simulink model "fixlib"  (Simulink 6.2)
settings: Solver=ode45  SolverMode=SingleTasking  StartTime=0.0  StopTime=10.0  RelTol=1e-3  AbsTol=1e-6
undefined symbols (not defined in the file or in its folder): k
settings Model: Creator=jacobs  LastModifiedBy=jacobs  ExtModeAutoUpdateStatusClock=off
settings DataIOCC: LimitDataPoints=off
settings OptimizationCC: BlockReduction=off  BooleanDataType=off
settings HardwareCC: TargetUnknown=on
settings GRTTargetCC: ModelReferenceCompliant=off  MatFileLogging=off

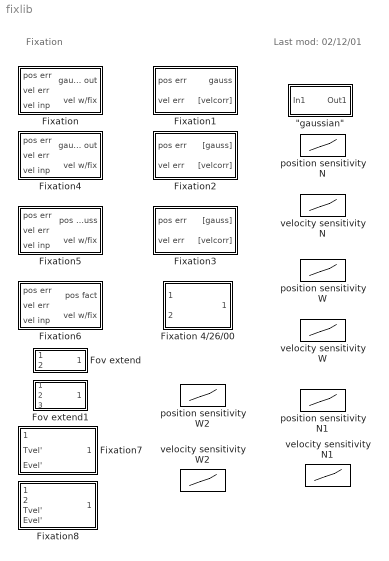
== system fixlib ==
  note: Last mod: 02/12/01
  note: Fixation
  "\"gaussian\"" : Subsystem
      mask Display: disp('"gaussian"')
  Fixation : Subsystem
  "Fixation 4/26/00 " : Subsystem
  Fixation1 : Subsystem
  Fixation2 : Subsystem
  Fixation3 : Subsystem
  Fixation4 : Subsystem
  Fixation5 : Subsystem
  Fixation6 : Subsystem
  Fixation7 : Subsystem
      mask Display: disp('Fixation')
  Fixation8 : Subsystem
      mask Display: disp('Fixation')
  Fov extend : Subsystem
      mask Display: disp('Fov Exten')
  Fov extend1 : Subsystem
      mask Display: disp('Fov Exten')
  position sensitivity N : Lookup  InputValues="[-5 -2  -1 -0.5   0.5   1    2    5]"  OutputValues="[  0    0   0.5   1      1   0.5   0   0 ]"  SaturateOnIntegerOverflow=on
  position sensitivity N1 : Lookup  InputValues="[-2  -1 -0.5 -0.25   0.25   0.5   1  2]"  OutputValues="[  0    0   .5   1      1   .5   0   0 ]"  SaturateOnIntegerOverflow=on
  position sensitivity W : Lookup  InputValues="[-5 -2  -1 -0.5   0.5   1    2    5]"  OutputValues="[ 0   0.5    1     1      1     1    0.5  0]"  SaturateOnIntegerOverflow=on
  position sensitivity W2 : Lookup  InputValues="[-5 -2  -1 -0.5   0.5   1    2    5]"  OutputValues="[ 0   0.125    0.5     1      1     0.5    0.125  0]"  SaturateOnIntegerOverflow=on
  velocity sensitivity N : Lookup  InputValues="[-30 -15   -8  -4   4     8  15  30]"  OutputValues="[  0      0      0.5    1   1  0.5   0   0 ]"  SaturateOnIntegerOverflow=on
  velocity sensitivity N1 : Lookup  InputValues="[-20 -16  -12   -6  -4  4   6   12  16 20]"  OutputValues="[0 0   0.1    0.3    1   1   0.3  0.1   0 0]"  SaturateOnIntegerOverflow=on
  velocity sensitivity W : Lookup  InputValues="[-30 -15   -8  -4   4     8  15  30]"  OutputValues="[0  0.5   1    1    1    1   0.5  0]"  SaturateOnIntegerOverflow=on
  velocity sensitivity W2 : Lookup  InputValues="[-30 -15   -8  -4   4     8  15  30]"  OutputValues="[0  0.125   0.5    1    1    0.5   0.125  0]"  SaturateOnIntegerOverflow=on

== system fixlib/"gaussian" ==
  note: calculates 1-e^(n*x*x) which is gaussian-like.
  In1 : Inport  Port=1  LatchInput=off
  Math Function : Math  SaturateOnIntegerOverflow=on
  Product : Product  Inputs=3  SaturateOnIntegerOverflow=on  RndMeth=Zero  InputSameDT=on
  n : Constant  Value=-1/4
  Out1 : Outport  InitialOutput=0
  wires:
  n/1 -> Product/3
  In1/1 -> Product/2, Product/1
  Product/1 -> Math Function/1
  Math Function/1 -> Out1/1

== system fixlib/Fixation ==
  note: This should have the effect of reducing the high velocity error (due
      | to CN oscillation or other sources) enough to permit an extension of
      | the foveation period.
  note: This factor is used (with an additional gain factor) to scale the velocity error,
      | which is then subtracted from the velocity signal that is sent from the
      | common neural integrator to the ocular motor neurons.
  note: Positional error is passed through a gaussian-like function whose greatest
      | response occurs between +/-0.5 deg (approx), corresponding to the sensitivity
      | of the fovea.
  note: Last mod: 04/19/00
  note: Fixation
  pos err : Inport  Port=1  LatchInput=off
  vel err : Inport  Port=2  LatchInput=off
  vel inp : Inport  Port=3  LatchInput=off
  "\"gaussian\"" : Subsystem
      mask Display: disp('"gaussian"')
  "\"gaussian\" gain" : Constant  Value=.5
  Product : Product  Inputs=3  SaturateOnIntegerOverflow=on  RndMeth=Zero  InputSameDT=on
  Sum : Sum  Inputs=-+  SaturateOnIntegerOverflow=on  InputSameDT=on
  gauss out : Outport  InitialOutput=0
  vel w/fix : Outport  Port=2  InitialOutput=0
  wires:
  "\"gaussian\" gain"/1 -> Product/2
  "\"gaussian\""/1(Out1) -> gauss out/1, Product/1
  pos err/1 -> "\"gaussian\""/1(In1)
  vel err/1 -> Product/3
  Product/1 -> Sum/1
  vel inp/1 -> Sum/2
  Sum/1 -> vel w/fix/1

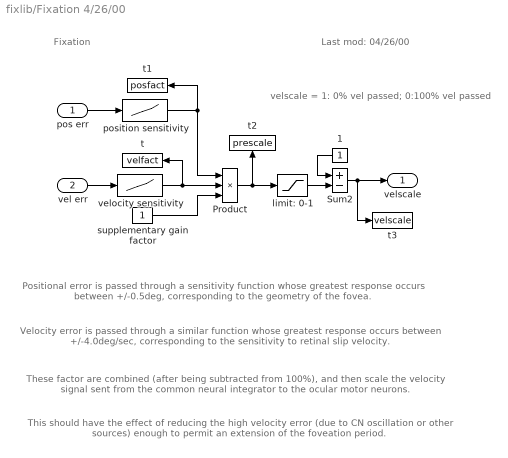
== system fixlib/Fixation 4/26/00  ==
  note: velscale =
      | 1: 0% vel passed;
      | 0:100% vel passed
  note: Velocity error is passed through a similar function whose greatest
      | response occurs between +/-4.0deg/sec, corresponding to the sensitivity
      | to retinal slip velocity.
  note: This should have the effect of reducing the high velocity error (due
      | to CN oscillation or other sources) enough to permit an extension of
      | the foveation period.
  note: These factor are combined (after being subtracted from 100%),
      | and then scale the velocity signal sent from the
      | common neural integrator to the ocular motor neurons.
  note: Positional error is passed through a sensitivity function whose greatest
      | response occurs between +/-0.5deg, corresponding to the geometry
      | of the fovea.
  note: Last mod: 04/26/00
  note: Fixation
  pos err : Inport  Port=1  LatchInput=off
  vel err : Inport  Port=2  LatchInput=off
  1 : Constant  Orientation=left
  Product : Product  Inputs=3  SaturateOnIntegerOverflow=on  RndMeth=Zero  InputSameDT=on
  Sum2 : Sum  Inputs=+-  SaturateOnIntegerOverflow=on  InputSameDT=on
  limit: 0-1 : Saturate  UpperLimit=1  LowerLimit=0
  position sensitivity : Lookup  InputValues="[-5 -2    -1  -0.5   0.5     1    2    5]"  OutputValues="[  0    0   0.25   1      1   0.25   0   0 ]"  SaturateOnIntegerOverflow=on
  supplementary gain factor : Constant
  t : ToWorkspace  VariableName=velfact  SaveFormat=Array
      mask init:
      | global t
      settings: MaxDataPoints=100000
  t1 : ToWorkspace  VariableName=posfact  SaveFormat=Array
      mask init:
      | global t
      settings: MaxDataPoints=100000
  t2 : ToWorkspace  VariableName=prescale  SaveFormat=Array
      mask init:
      | global t
      settings: Orientation=up  MaxDataPoints=100000
  t3 : ToWorkspace  VariableName=velscale  SaveFormat=Array
      mask init:
      | global t
      settings: MaxDataPoints=100000
  velocity sensitivity : Lookup  InputValues="[-30 -15    -8   -4    4     8    15  30]"  OutputValues="[  0      0      0.25    1   1  0.25   0   0 ]"  SaturateOnIntegerOverflow=on
  velscale : Outport  InitialOutput=0
  wires:
  Sum2/1 -> t3/1, velscale/1
  limit: 0-1/1 -> Sum2/2
  1/1 -> Sum2/1
  position sensitivity/1 -> Product/1, t1/1
  pos err/1 -> position sensitivity/1
  Product/1 -> limit: 0-1/1, t2/1
  velocity sensitivity/1 -> t/1, Product/2
  supplementary gain factor/1 -> Product/3
  vel err/1 -> velocity sensitivity/1

== system fixlib/Fixation1 ==
  note: velocity
      | correction
  note: This should have the effect of reducing the high velocity error (due
      | to CN oscillation or other sources) enough to permit an extension of
      | the foveation period.
  note: This factor is used (with an additional gain factor) to scale the velocity error,
      | which will then subtracted from the velocity signal that is sent from the
      | common neural integrator to the ocular motor neurons.
  note: Positional error is passed through a gaussian-like function whose greatest
      | response occurs between +/-0.5 deg (approx), corresponding to the sensitivity
      | of the fovea.
  note: Last mod: 04/19/00
  note: Fixation
  pos err : Inport  Port=1  LatchInput=off
  vel err : Inport  Port=2  LatchInput=off
  "\"gaussian\"" : Subsystem
      mask Display: disp('"gaussian"')
  "\"gaussian\" gain" : Constant  Value=.5
  Product : Product  Inputs=3  SaturateOnIntegerOverflow=on  RndMeth=Zero  InputSameDT=on
  To Workspace30 : ToWorkspace  VariableName=velcorr  SaveFormat=Array
      settings: MaxDataPoints=10000
  gauss : Outport  InitialOutput=0
  "[velcorr]" : Outport  Port=2  InitialOutput=0
  wires:
  Product/1 -> To Workspace30/1, "[velcorr]"/1
  "\"gaussian\" gain"/1 -> Product/2
  "\"gaussian\""/1(Out1) -> gauss/1, Product/1
  pos err/1 -> "\"gaussian\""/1(In1)
  vel err/1 -> Product/3

== system fixlib/Fixation2 ==
  note: [tpstar]
  note: [svpr]
  note: velocity
      | correction
  note: This should have the effect of reducing the high velocity error (due
      | to CN oscillation or other sources) enough to permit an extension of
      | the foveation period.
  note: This factor is used (with an additional gain factor) to scale the velocity error,
      | which will then subtracted from the velocity signal that is sent from the
      | common neural integrator to the ocular motor neurons.
  note: Positional error is passed through a gaussian-like function whose greatest
      | response occurs between +/-0.5 deg (approx), corresponding to the sensitivity
      | of the fovea.
  note: Last mod: 04/21/00
  note: Fixation
  pos err : Inport  Port=1  LatchInput=off
  vel err : Inport  Port=2  LatchInput=off
  "\"gaussian\"" : Subsystem
      mask Display: disp('"gaussian"')
  "\"gaussian\" gain" : Constant  Value=.5
  Product : Product  Inputs=3  SaturateOnIntegerOverflow=on  RndMeth=Zero  InputSameDT=on
  Product1 : Product  SaturateOnIntegerOverflow=on  RndMeth=Zero  InputSameDT=on
  To Workspace30 : ToWorkspace  VariableName=velcorr  SaveFormat=Array
      settings: MaxDataPoints=10000
  k : Constant  Value=k
  "[gauss]" : Outport  InitialOutput=0
  "[velcorr]" : Outport  Port=2  InitialOutput=0
  wires:
  k/1 -> Product/3
  Product/1 -> To Workspace30/1, "[velcorr]"/1
  Product1/1 -> Product/1, "[gauss]"/1
  "\"gaussian\" gain"/1 -> Product1/2
  "\"gaussian\""/1(Out1) -> Product1/1
  pos err/1 -> "\"gaussian\""/1(In1)
  vel err/1 -> Product/2

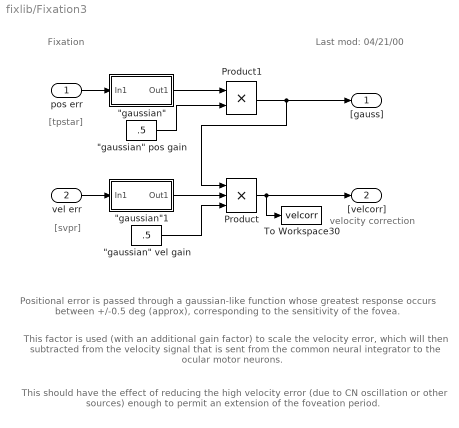
== system fixlib/Fixation3 ==
  note: [tpstar]
  note: [svpr]
  note: velocity
      | correction
  note: This should have the effect of reducing the high velocity error (due
      | to CN oscillation or other sources) enough to permit an extension of
      | the foveation period.
  note: This factor is used (with an additional gain factor) to scale the velocity error,
      | which will then subtracted from the velocity signal that is sent from the
      | common neural integrator to the ocular motor neurons.
  note: Positional error is passed through a gaussian-like function whose greatest
      | response occurs between +/-0.5 deg (approx), corresponding to the sensitivity
      | of the fovea.
  note: Last mod: 04/21/00
  note: Fixation
  pos err : Inport  Port=1  LatchInput=off
  vel err : Inport  Port=2  LatchInput=off
  "\"gaussian\"" : Subsystem
      mask Display: disp('"gaussian"')
  "\"gaussian\" pos gain" : Constant  Value=.5
  "\"gaussian\" vel gain" : Constant  Value=.5
  "\"gaussian\"1" : Subsystem
      mask Display: disp('"gaussian"')
  Product : Product  Inputs=3  SaturateOnIntegerOverflow=on  RndMeth=Zero  InputSameDT=on
  Product1 : Product  SaturateOnIntegerOverflow=on  RndMeth=Zero  InputSameDT=on
  To Workspace30 : ToWorkspace  VariableName=velcorr  SaveFormat=Array
      settings: MaxDataPoints=10000
  "[gauss]" : Outport  InitialOutput=0
  "[velcorr]" : Outport  Port=2  InitialOutput=0
  wires:
  "\"gaussian\" vel gain"/1 -> Product/3
  Product/1 -> To Workspace30/1, "[velcorr]"/1
  "\"gaussian\"1"/1(Out1) -> Product/2
  vel err/1 -> "\"gaussian\"1"/1(In1)
  Product1/1 -> Product/1, "[gauss]"/1
  "\"gaussian\" pos gain"/1 -> Product1/2
  "\"gaussian\""/1(Out1) -> Product1/1
  pos err/1 -> "\"gaussian\""/1(In1)

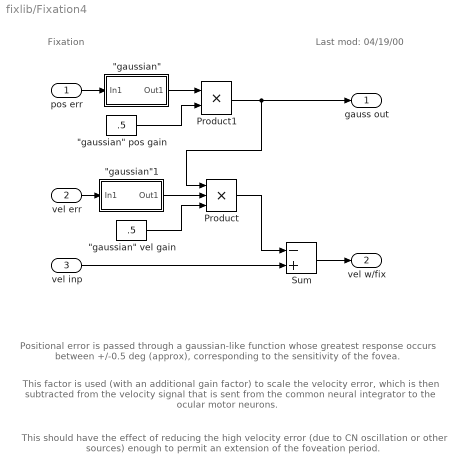
== system fixlib/Fixation4 ==
  note: This should have the effect of reducing the high velocity error (due
      | to CN oscillation or other sources) enough to permit an extension of
      | the foveation period.
  note: This factor is used (with an additional gain factor) to scale the velocity error,
      | which is then subtracted from the velocity signal that is sent from the
      | common neural integrator to the ocular motor neurons.
  note: Positional error is passed through a gaussian-like function whose greatest
      | response occurs between +/-0.5 deg (approx), corresponding to the sensitivity
      | of the fovea.
  note: Last mod: 04/19/00
  note: Fixation
  pos err : Inport  Port=1  LatchInput=off
  vel err : Inport  Port=2  LatchInput=off
  vel inp : Inport  Port=3  LatchInput=off
  "\"gaussian\"" : Subsystem
      mask Display: disp('"gaussian"')
  "\"gaussian\" pos gain" : Constant  Value=.5
  "\"gaussian\" vel gain" : Constant  Value=.5
  "\"gaussian\"1" : Subsystem
      mask Display: disp('"gaussian"')
  Product : Product  Inputs=3  SaturateOnIntegerOverflow=on  RndMeth=Zero  InputSameDT=on
  Product1 : Product  SaturateOnIntegerOverflow=on  RndMeth=Zero  InputSameDT=on
  Sum : Sum  Inputs=-+  SaturateOnIntegerOverflow=on  InputSameDT=on
  gauss out : Outport  InitialOutput=0
  vel w/fix : Outport  Port=2  InitialOutput=0
  wires:
  "\"gaussian\" vel gain"/1 -> Product/3
  vel inp/1 -> Sum/2
  Sum/1 -> vel w/fix/1
  "\"gaussian\"1"/1(Out1) -> Product/2
  vel err/1 -> "\"gaussian\"1"/1(In1)
  Product1/1 -> Product/1, gauss out/1
  "\"gaussian\" pos gain"/1 -> Product1/2
  "\"gaussian\""/1(Out1) -> Product1/1
  Product/1 -> Sum/1
  pos err/1 -> "\"gaussian\""/1(In1)

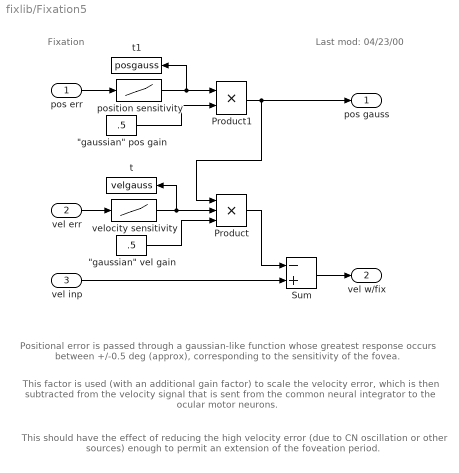
== system fixlib/Fixation5 ==
  note: This should have the effect of reducing the high velocity error (due
      | to CN oscillation or other sources) enough to permit an extension of
      | the foveation period.
  note: This factor is used (with an additional gain factor) to scale the velocity error,
      | which is then subtracted from the velocity signal that is sent from the
      | common neural integrator to the ocular motor neurons.
  note: Positional error is passed through a gaussian-like function whose greatest
      | response occurs between +/-0.5 deg (approx), corresponding to the sensitivity
      | of the fovea.
  note: Last mod: 04/23/00
  note: Fixation
  pos err : Inport  Port=1  LatchInput=off
  vel err : Inport  Port=2  LatchInput=off
  vel inp : Inport  Port=3  LatchInput=off
  "\"gaussian\" pos gain" : Constant  Value=.5
  "\"gaussian\" vel gain" : Constant  Value=.5
  Product : Product  Inputs=3  SaturateOnIntegerOverflow=on  RndMeth=Zero  InputSameDT=on
  Product1 : Product  SaturateOnIntegerOverflow=on  RndMeth=Zero  InputSameDT=on
  Sum : Sum  Inputs=-+  SaturateOnIntegerOverflow=on  InputSameDT=on
  position sensitivity : Lookup  InputValues="[-5 -2  -1 -0.5   0.5   1    2    5]"  OutputValues="[  0    0   0.5   1      1   0.5   0   0 ]"  SaturateOnIntegerOverflow=on
  t : ToWorkspace  VariableName=velgauss  SaveFormat=Array
      mask init:
      | global t
      settings: MaxDataPoints=100000
  t1 : ToWorkspace  VariableName=posgauss  SaveFormat=Array
      mask init:
      | global t
      settings: MaxDataPoints=100000
  velocity sensitivity : Lookup  InputValues="[-30 -15   -8  -4   4     8  15  30]"  OutputValues="[  0      0      0.5    1   1  0.5   0   0 ]"  SaturateOnIntegerOverflow=on
  pos gauss : Outport  InitialOutput=0
  vel w/fix : Outport  Port=2  InitialOutput=0
  wires:
  position sensitivity/1 -> t1/1, Product1/1
  velocity sensitivity/1 -> t/1, Product/2
  "\"gaussian\" vel gain"/1 -> Product/3
  vel inp/1 -> Sum/2
  Sum/1 -> vel w/fix/1
  vel err/1 -> velocity sensitivity/1
  Product/1 -> Sum/1
  Product1/1 -> Product/1, pos gauss/1
  "\"gaussian\" pos gain"/1 -> Product1/2
  pos err/1 -> position sensitivity/1

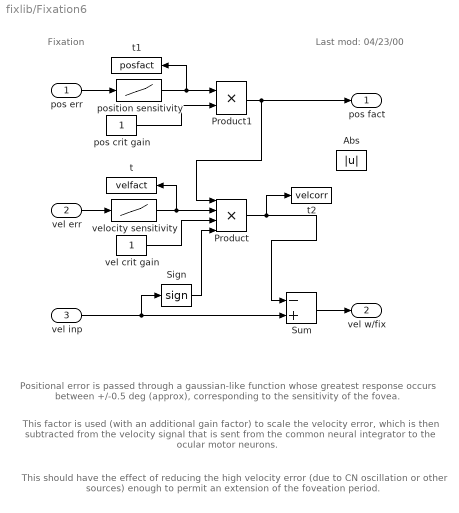
== system fixlib/Fixation6 ==
  note: This should have the effect of reducing the high velocity error (due
      | to CN oscillation or other sources) enough to permit an extension of
      | the foveation period.
  note: This factor is used (with an additional gain factor) to scale the velocity error,
      | which is then subtracted from the velocity signal that is sent from the
      | common neural integrator to the ocular motor neurons.
  note: Positional error is passed through a gaussian-like function whose greatest
      | response occurs between +/-0.5 deg (approx), corresponding to the sensitivity
      | of the fovea.
  note: Last mod: 04/23/00
  note: Fixation
  pos err : Inport  Port=1  LatchInput=off
  vel err : Inport  Port=2  LatchInput=off
  vel inp : Inport  Port=3  LatchInput=off
  Abs : Abs  SaturateOnIntegerOverflow=on
  Product : Product  Inputs=4  SaturateOnIntegerOverflow=on  RndMeth=Zero  InputSameDT=on
  Product1 : Product  SaturateOnIntegerOverflow=on  RndMeth=Zero  InputSameDT=on
  Sign : Signum
  Sum : Sum  Inputs=-+  SaturateOnIntegerOverflow=on  InputSameDT=on
  pos crit gain : Constant
  position sensitivity : Lookup  InputValues="[-5 -2  -1 -0.5   0.5   1    2    5]"  OutputValues="[  0    0   0.5   1      1   0.5   0   0 ]"  SaturateOnIntegerOverflow=on
  t : ToWorkspace  VariableName=velfact  SaveFormat=Array
      mask init:
      | global t
      settings: MaxDataPoints=100000
  t1 : ToWorkspace  VariableName=posfact  SaveFormat=Array
      mask init:
      | global t
      settings: MaxDataPoints=100000
  t2 : ToWorkspace  VariableName=velcorr  SaveFormat=Array
      mask init:
      | global t
      settings: MaxDataPoints=100000
  vel crit gain : Constant
  velocity sensitivity : Lookup  InputValues="[-30 -15   -8  -4   4     8  15  30]"  OutputValues="[  0      0      0.5    1   1  0.5   0   0 ]"  SaturateOnIntegerOverflow=on
  pos fact : Outport  InitialOutput=0
  vel w/fix : Outport  Port=2  InitialOutput=0
  wires:
  Product/1 -> t2/1, Sum/1
  Sign/1 -> Product/4
  vel inp/1 -> Sign/1, Sum/2
  Sum/1 -> vel w/fix/1
  position sensitivity/1 -> t1/1, Product1/1
  velocity sensitivity/1 -> t/1, Product/2
  vel crit gain/1 -> Product/3
  vel err/1 -> velocity sensitivity/1
  Product1/1 -> Product/1, pos fact/1
  pos crit gain/1 -> Product1/2
  pos err/1 -> position sensitivity/1

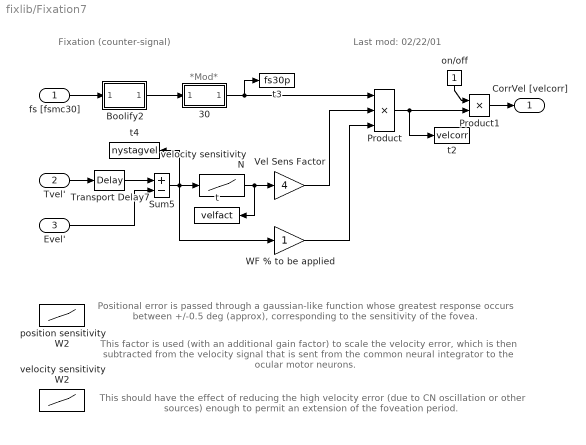
== system fixlib/Fixation7 ==
  note: *Mod*
  note: This should have the effect of reducing the high velocity error (due
      | to CN oscillation or other sources) enough to permit an extension of
      | the foveation period.
  note: This factor is used (with an additional gain factor) to scale the velocity error,
      | which is then subtracted from the velocity signal that is sent from the
      | common neural integrator to the ocular motor neurons.
  note: Positional error is passed through a gaussian-like function whose greatest
      | response occurs between +/-0.5 deg (approx), corresponding to the sensitivity
      | of the fovea.
  note: Last mod: 02/22/01
  note: Fixation (counter-signal)
  fs [fsmc30] : Inport  Port=1  LatchInput=off
  Tvel' : Inport  Port=2  LatchInput=off
  Evel' : Inport  Port=3  LatchInput=off
  "30 " : Subsystem  mask{prolong=30}
      mask prompts: prolong "Prolong pulse by?  (msec)"
      mask Display: disp('prolong')
  Boolify2 : Subsystem
      mask Display: disp('Boolify')
  Product : Product  Inputs=3  SaturateOnIntegerOverflow=on  RndMeth=Zero  InputSameDT=on
  Product1 : Product  SaturateOnIntegerOverflow=on  RndMeth=Zero  InputSameDT=on
  Sum5 : Sum  Inputs=+-  SaturateOnIntegerOverflow=on  InputSameDT=on
  Transport Delay7 : TransportDelay  DelayTime=0.050
      mask Display: disp('50ms')
  Vel Sens Factor : Gain  Gain=4  SaturateOnIntegerOverflow=on
  WF % to be applied : Gain  SaturateOnIntegerOverflow=on
  on/off : Constant  Orientation=down
  position sensitivity W2 : Lookup  InputValues="[-5 -2  -1 -0.5   0.5   1    2    5]"  OutputValues="[ 0   0.125    0.5     1      1     0.5    0.125  0]"  SaturateOnIntegerOverflow=on
  t : ToWorkspace  VariableName=velfact  SaveFormat=Array
      mask init:
      | global t
      settings: MaxDataPoints=100000
  t2 : ToWorkspace  VariableName=velcorr  SaveFormat=Array
      mask init:
      | global t
      settings: MaxDataPoints=100000
  t3 : ToWorkspace  VariableName=fs30p  SaveFormat=Array
      mask init:
      | global t
      settings: MaxDataPoints=100000
  t4 : ToWorkspace  VariableName=nystagvel  SaveFormat=Array
      mask init:
      | global t
      settings: MaxDataPoints=100000
  velocity sensitivity N : Lookup  InputValues="[-20 -16  -12   -6  -4  4   6   12  16 20]"  OutputValues="[0 0   0.1    0.3    1   1   0.3  0.1   0 0]"  SaturateOnIntegerOverflow=on
  velocity sensitivity W2 : Lookup  InputValues="[-30 -15   -8  -4   4     8  15  30]"  OutputValues="[0  0.125   0.5    1    1    0.5   0.125  0]"  SaturateOnIntegerOverflow=on
  " CorrVel [velcorr]" : Outport  InitialOutput=0
  wires:
  Vel Sens Factor/1 -> Product/2
  "30 "/1(value(out)) -> t3/1, Product/1
  Boolify2/1(Out1) -> "30 "/1(value(in))
  fs [fsmc30]/1 -> Boolify2/1(In1)
  on/off/1 -> Product1/1
  Product1/1 -> " CorrVel [velcorr]"/1
  Product/1 -> Product1/2, t2/1
  WF % to be applied/1 -> Product/3
  Transport Delay7/1 -> Sum5/1
  Tvel'/1 -> Transport Delay7/1
  Evel'/1 -> Sum5/2
  velocity sensitivity N/1 -> t/1, Vel Sens Factor/1
  Sum5/1 -> WF % to be applied/1, t4/1, velocity sensitivity N/1

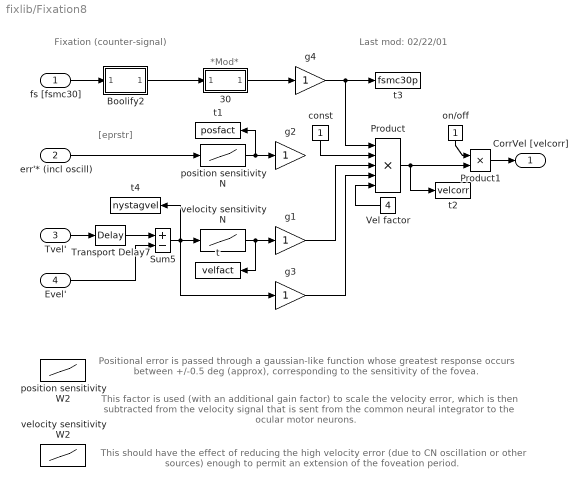
== system fixlib/Fixation8 ==
  note: Fixation (counter-signal)
  note: Last mod: 02/22/01
  note: Positional error is passed through a gaussian-like function whose greatest
      | response occurs between +/-0.5 deg (approx), corresponding to the sensitivity
      | of the fovea.
  note: This factor is used (with an additional gain factor) to scale the velocity error,
      | which is then subtracted from the velocity signal that is sent from the
      | common neural integrator to the ocular motor neurons.
  note: This should have the effect of reducing the high velocity error (due
      | to CN oscillation or other sources) enough to permit an extension of
      | the foveation period.
  note: [eprstr]
  note: *Mod*
  fs [fsmc30] : Inport  Port=1  LatchInput=off
  err'* (incl oscill) : Inport  Port=2  LatchInput=off
  Tvel' : Inport  Port=3  LatchInput=off
  Evel' : Inport  Port=4  LatchInput=off
  "30 " : Subsystem  mask{prolong=30}
      mask prompts: prolong "Prolong pulse by?  (msec)"
      mask Display: disp('prolong')
  Boolify2 : Subsystem
      mask Display: disp('Boolify')
  Product : Product  Inputs=5  SaturateOnIntegerOverflow=on  RndMeth=Zero  InputSameDT=on
  Product1 : Product  SaturateOnIntegerOverflow=on  RndMeth=Zero  InputSameDT=on
  Sum5 : Sum  Inputs=+-  SaturateOnIntegerOverflow=on  InputSameDT=on
  Transport Delay7 : TransportDelay  DelayTime=0.050
      mask Display: disp('50ms')
  Vel factor : Constant  Orientation=left  Value=4
  const : Constant  Orientation=down
  g{1..4} (4 alike) : Gain  SaturateOnIntegerOverflow=on
  on/off : Constant  Orientation=down
  position sensitivity N : Lookup  InputValues="[-2  -1 -0.5 -0.25   0.25   0.5   1  2]"  OutputValues="[  0    0   .5   1      1   .5   0   0 ]"  SaturateOnIntegerOverflow=on
  position sensitivity W2 : Lookup  InputValues="[-5 -2  -1 -0.5   0.5   1    2    5]"  OutputValues="[ 0   0.125    0.5     1      1     0.5    0.125  0]"  SaturateOnIntegerOverflow=on
  t : ToWorkspace  VariableName=velfact  SaveFormat=Array
      mask init:
      | global t
      settings: MaxDataPoints=100000
  t1 : ToWorkspace  VariableName=posfact  SaveFormat=Array
      mask init:
      | global t
      settings: MaxDataPoints=100000
  t2 : ToWorkspace  VariableName=velcorr  SaveFormat=Array
      mask init:
      | global t
      settings: MaxDataPoints=100000
  t3 : ToWorkspace  VariableName=fsmc30p  SaveFormat=Array
      mask init:
      | global t
      settings: MaxDataPoints=100000
  t4 : ToWorkspace  VariableName=nystagvel  SaveFormat=Array
      mask init:
      | global t
      settings: MaxDataPoints=100000
  velocity sensitivity N : Lookup  InputValues="[-20 -16  -12   -6  -4  4   6   12  16 20]"  OutputValues="[0 0   0.1    0.3    1   1   0.3  0.1   0 0]"  SaturateOnIntegerOverflow=on
  velocity sensitivity W2 : Lookup  InputValues="[-30 -15   -8  -4   4     8  15  30]"  OutputValues="[0  0.125   0.5    1    1    0.5   0.125  0]"  SaturateOnIntegerOverflow=on
  " CorrVel [velcorr]" : Outport  InitialOutput=0
  wires:
  Sum5/1 -> velocity sensitivity N/1, t4/1, g3/1
  velocity sensitivity N/1 -> g1/1, t/1
  Evel'/1 -> Sum5/2
  Tvel'/1 -> Transport Delay7/1
  Transport Delay7/1 -> Sum5/1
  position sensitivity N/1 -> g2/1, t1/1
  g3/1 -> Product/4
  g1/1 -> Product/3
  Product/1 -> t2/1, Product1/2
  Product1/1 -> " CorrVel [velcorr]"/1
  on/off/1 -> Product1/1
  Vel factor/1 -> Product/5
  g4/1 -> Product/1, t3/1
  fs [fsmc30]/1 -> Boolify2/1(In1)
  "30 "/1(value(out)) -> g4/1
  const/1 -> Product/2
  Boolify2/1(Out1) -> "30 "/1(value(in))
  err'* (incl oscill)/1 -> position sensitivity N/1

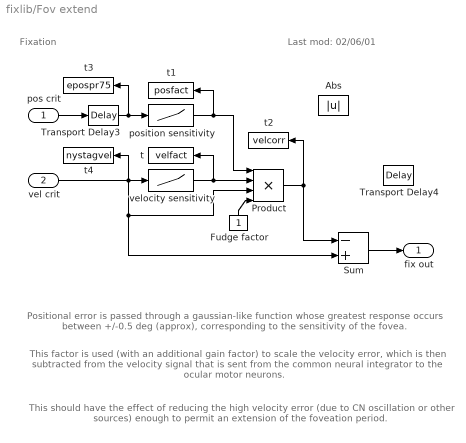
== system fixlib/Fov extend ==
  note: This should have the effect of reducing the high velocity error (due
      | to CN oscillation or other sources) enough to permit an extension of
      | the foveation period.
  note: This factor is used (with an additional gain factor) to scale the velocity error,
      | which is then subtracted from the velocity signal that is sent from the
      | common neural integrator to the ocular motor neurons.
  note: Positional error is passed through a gaussian-like function whose greatest
      | response occurs between +/-0.5 deg (approx), corresponding to the sensitivity
      | of the fovea.
  note: Last mod: 02/06/01
  note: Fixation
  pos crit : Inport  Port=1  LatchInput=off
  vel crit : Inport  Port=2  LatchInput=off
  Abs : Abs  SaturateOnIntegerOverflow=on
  Fudge factor : Constant  Orientation=up
  Product : Product  Inputs=4  SaturateOnIntegerOverflow=on  RndMeth=Zero  InputSameDT=on
  Sum : Sum  Inputs=-+  SaturateOnIntegerOverflow=on  InputSameDT=on
  Transport Delay3 : TransportDelay  DelayTime=0.075
      mask Display: disp('75ms')
  Transport Delay4 : TransportDelay  DelayTime=0.001
      mask Display: disp('1ms')
  position sensitivity : Lookup  InputValues="[-5 -2  -1 -0.5   0.5   1    2    5]"  OutputValues="[  0    0   0.5   1      1   0.5   0   0 ]"  SaturateOnIntegerOverflow=on
  t : ToWorkspace  VariableName=velfact  SaveFormat=Array
      mask init:
      | global t
      settings: MaxDataPoints=100000
  t1 : ToWorkspace  VariableName=posfact  SaveFormat=Array
      mask init:
      | global t
      settings: MaxDataPoints=100000
  t2 : ToWorkspace  VariableName=velcorr  SaveFormat=Array
      mask init:
      | global t
      settings: MaxDataPoints=100000
  t3 : ToWorkspace  VariableName=epospr75  SaveFormat=Array
      mask init:
      | global t
      settings: MaxDataPoints=100000
  t4 : ToWorkspace  VariableName=nystagvel  SaveFormat=Array
      mask init:
      | global t
      settings: MaxDataPoints=100000
  velocity sensitivity : Lookup  InputValues="[-30 -15   -8  -4   4     8  15  30]"  OutputValues="[  0      0      0.5    1   1  0.5   0   0 ]"  SaturateOnIntegerOverflow=on
  fix out : Outport  InitialOutput=0
  wires:
  Product/1 -> Sum/1, t2/1
  Fudge factor/1 -> Product/4
  Sum/1 -> fix out/1
  Transport Delay3/1 -> t3/1, position sensitivity/1
  pos crit/1 -> Transport Delay3/1
  vel crit/1 -> Product/3, Sum/2, t4/1, velocity sensitivity/1
  position sensitivity/1 -> Product/1, t1/1
  velocity sensitivity/1 -> t/1, Product/2

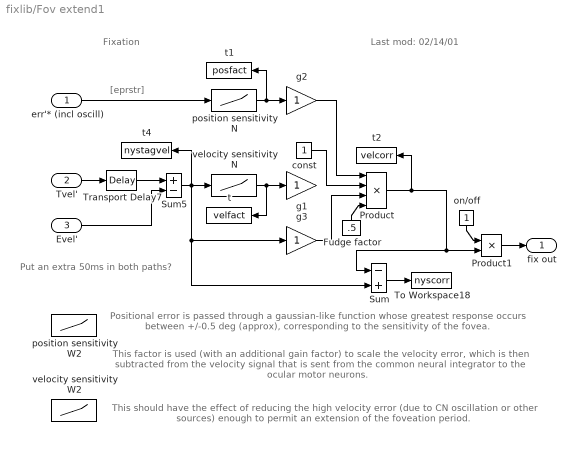
== system fixlib/Fov extend1 ==
  note: Fixation
  note: Last mod: 02/14/01
  note: Positional error is passed through a gaussian-like function whose greatest
      | response occurs between +/-0.5 deg (approx), corresponding to the sensitivity
      | of the fovea.
  note: This factor is used (with an additional gain factor) to scale the velocity error,
      | which is then subtracted from the velocity signal that is sent from the
      | common neural integrator to the ocular motor neurons.
  note: This should have the effect of reducing the high velocity error (due
      | to CN oscillation or other sources) enough to permit an extension of
      | the foveation period.
  note: Put an extra 50ms
      | in both paths?
  note: [eprstr]
  err'* (incl oscill) : Inport  Port=1  LatchInput=off
  Tvel' : Inport  Port=2  LatchInput=off
  Evel' : Inport  Port=3  LatchInput=off
  Fudge factor : Constant  Orientation=up  Value=.5
  Product : Product  Inputs=4  SaturateOnIntegerOverflow=on  RndMeth=Zero  InputSameDT=on
  Product1 : Product  SaturateOnIntegerOverflow=on  RndMeth=Zero  InputSameDT=on
  Sum : Sum  Inputs=-+  SaturateOnIntegerOverflow=on  InputSameDT=on
  Sum5 : Sum  Inputs=+-  SaturateOnIntegerOverflow=on  InputSameDT=on
  To Workspace18 : ToWorkspace  VariableName=nyscorr  SaveFormat=Array
      settings: MaxDataPoints=10000
  Transport Delay7 : TransportDelay  DelayTime=0.050
      mask Display: disp('50ms')
  const : Constant
  g1 : Gain  SaturateOnIntegerOverflow=on
  g2 : Gain  SaturateOnIntegerOverflow=on
  g3 : Gain  SaturateOnIntegerOverflow=on
  on/off : Constant  Orientation=down
  position sensitivity N : Lookup  InputValues="[-5 -2  -1 -0.5   0.5   1    2    5]"  OutputValues="[  0    0   0.25   1      1   0.25   0   0 ]"  SaturateOnIntegerOverflow=on
  position sensitivity W2 : Lookup  InputValues="[-5 -2  -1 -0.5   0.5   1    2    5]"  OutputValues="[ 0   0.125    0.5     1      1     0.5    0.125  0]"  SaturateOnIntegerOverflow=on
  t : ToWorkspace  VariableName=velfact  SaveFormat=Array
      mask init:
      | global t
      settings: MaxDataPoints=100000
  t1 : ToWorkspace  VariableName=posfact  SaveFormat=Array
      mask init:
      | global t
      settings: MaxDataPoints=100000
  t2 : ToWorkspace  VariableName=velcorr  SaveFormat=Array
      mask init:
      | global t
      settings: MaxDataPoints=100000
  t4 : ToWorkspace  VariableName=nystagvel  SaveFormat=Array
      mask init:
      | global t
      settings: MaxDataPoints=100000
  velocity sensitivity N : Lookup  InputValues="[-30 -15   -6  -4   4     6  15  30]"  OutputValues="[  0      0      1    1   1  1   0   0 ]"  SaturateOnIntegerOverflow=on
  velocity sensitivity W2 : Lookup  InputValues="[-30 -15   -8  -4   4     8  15  30]"  OutputValues="[0  0.125   0.5    1    1    0.5   0.125  0]"  SaturateOnIntegerOverflow=on
  fix out : Outport  InitialOutput=0
  wires:
  Fudge factor/1 -> Product/4
  Product/1 -> t2/1, Product1/2, Sum/1
  g3/1 -> Product/3
  Sum5/1 -> velocity sensitivity N/1, t4/1, g3/1, Sum/2
  velocity sensitivity N/1 -> g1/1, t/1
  Evel'/1 -> Sum5/2
  Tvel'/1 -> Transport Delay7/1
  Transport Delay7/1 -> Sum5/1
  Sum/1 -> To Workspace18/1
  Product1/1 -> fix out/1
  on/off/1 -> Product1/1
  err'* (incl oscill)/1 -> position sensitivity N/1
  g2/1 -> Product/1
  position sensitivity N/1 -> g2/1, t1/1
  const/1 -> Product/2

== system fixlib/Fixation/"gaussian" ==
  note: calculates 1-e^(n*x*x) which is gaussian-like.
  In1 : Inport  Port=1  LatchInput=off
  Math Function : Math  SaturateOnIntegerOverflow=on
  Product : Product  Inputs=3  SaturateOnIntegerOverflow=on  RndMeth=Zero  InputSameDT=on
  n : Constant  Value=-1/4
  Out1 : Outport  InitialOutput=0
  wires:
  Math Function/1 -> Out1/1
  Product/1 -> Math Function/1
  In1/1 -> Product/1, Product/2
  n/1 -> Product/3

== system fixlib/Fixation1/"gaussian" ==
  note: calculates 1-e^(n*x*x) which is gaussian-like.
  In1 : Inport  Port=1  LatchInput=off
  Math Function : Math  SaturateOnIntegerOverflow=on
  Product : Product  Inputs=3  SaturateOnIntegerOverflow=on  RndMeth=Zero  InputSameDT=on
  n : Constant  Value=-1/4
  Out1 : Outport  InitialOutput=0
  wires:
  Math Function/1 -> Out1/1
  Product/1 -> Math Function/1
  In1/1 -> Product/1, Product/2
  n/1 -> Product/3

== system fixlib/Fixation2/"gaussian" ==
  note: calculates 1-e^(n*x*x) which is gaussian-like.
  In1 : Inport  Port=1  LatchInput=off
  Math Function : Math  SaturateOnIntegerOverflow=on
  Product : Product  Inputs=3  SaturateOnIntegerOverflow=on  RndMeth=Zero  InputSameDT=on
  n : Constant  Value=-1/4
  Out1 : Outport  InitialOutput=0
  wires:
  Math Function/1 -> Out1/1
  Product/1 -> Math Function/1
  In1/1 -> Product/1, Product/2
  n/1 -> Product/3

== system fixlib/Fixation3/"gaussian" ==
  note: calculates 1-e^(n*x*x) which is gaussian-like.
  In1 : Inport  Port=1  LatchInput=off
  Math Function : Math  SaturateOnIntegerOverflow=on
  Product : Product  Inputs=3  SaturateOnIntegerOverflow=on  RndMeth=Zero  InputSameDT=on
  n : Constant  Value=-1/4
  Out1 : Outport  InitialOutput=0
  wires:
  Math Function/1 -> Out1/1
  Product/1 -> Math Function/1
  In1/1 -> Product/1, Product/2
  n/1 -> Product/3

== system fixlib/Fixation3/"gaussian"1 ==
  note: calculates 1-e^(n*x*x) which is gaussian-like.
  In1 : Inport  Port=1  LatchInput=off
  Math Function : Math  SaturateOnIntegerOverflow=on
  Product : Product  Inputs=3  SaturateOnIntegerOverflow=on  RndMeth=Zero  InputSameDT=on
  n : Constant  Value=-1/4
  Out1 : Outport  InitialOutput=0
  wires:
  n/1 -> Product/3
  In1/1 -> Product/2, Product/1
  Product/1 -> Math Function/1
  Math Function/1 -> Out1/1

== system fixlib/Fixation4/"gaussian" ==
  note: calculates 1-e^(n*x*x) which is gaussian-like.
  In1 : Inport  Port=1  LatchInput=off
  Math Function : Math  SaturateOnIntegerOverflow=on
  Product : Product  Inputs=3  SaturateOnIntegerOverflow=on  RndMeth=Zero  InputSameDT=on
  n : Constant  Value=-1/4
  Out1 : Outport  InitialOutput=0
  wires:
  Math Function/1 -> Out1/1
  Product/1 -> Math Function/1
  In1/1 -> Product/1, Product/2
  n/1 -> Product/3

== system fixlib/Fixation4/"gaussian"1 ==
  note: calculates 1-e^(n*x*x) which is gaussian-like.
  In1 : Inport  Port=1  LatchInput=off
  Math Function : Math  SaturateOnIntegerOverflow=on
  Product : Product  Inputs=3  SaturateOnIntegerOverflow=on  RndMeth=Zero  InputSameDT=on
  n : Constant  Value=-1/4
  Out1 : Outport  InitialOutput=0
  wires:
  Math Function/1 -> Out1/1
  Product/1 -> Math Function/1
  In1/1 -> Product/1, Product/2
  n/1 -> Product/3

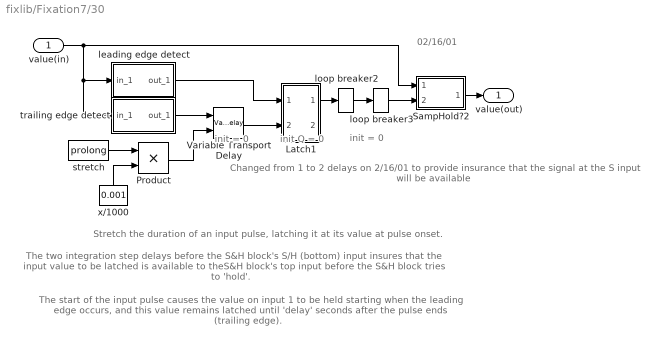
== system fixlib/Fixation7/30  ==
  note: Changed from 1 to 2 delays
      | on 2/16/01 to provide insurance that
      | the signal at the S input will be available
  note: init Q = 0
  note: Stretch the duration of an input pulse, latching it at its value at pulse onset.
  note: The two integration step delays before the S&H block's S/H (bottom) input insures
      | that the input value to be latched is available to theS&H block's top input
      | before the S&H block tries to 'hold'.
  note: The start of the input pulse causes the value on input 1 to be held starting when the leading
      | edge occurs, and this value remains latched until 'delay' seconds after the pulse ends (trailing edge).
  note: 02/16/01
  note: init = 0
  note: init = 0
  value(in) : Inport  Port=1  LatchInput=off
  " x/1000" : Constant  Orientation=up  Value=0.001
  Latch1 : Subsystem  mask(Latch){@1=0}
      mask prompts: @1 "Initial State for Output "Q":"
      mask help: Latch
      mask init:
      | ini=(@1~=0);
      mask Help: Latches the S input.  When S (set) is one, the Q output  becomes one.  The output remains one until the R (reset) input becomes one, forcing the output to zero.  If both R and S are one, the latch will be in an undefined state.
      mask Display: disp('S   Q\n\nR  !Q')
  Product : Product  SaturateOnIntegerOverflow=on  RndMeth=Zero  InputSameDT=on
  SampHold?2 : Subsystem
      mask Display: disp('S=L\nH=H')
  Variable Transport Delay : VariableTransportDelay  MaximumDelay=10
  leading edge detect : Subsystem
      mask Display: disp('Leading\nEdge Det')
  loop breaker2 : Memory
  loop breaker3 : Memory
  stretch : Constant  Value=prolong
  trailing edge detect : Subsystem
      mask Display: disp('Trailing\nEdge Det')
  value(out) : Outport  InitialOutput=0
  wires:
  Variable Transport Delay/1 -> Latch1/2(in_2)
  leading edge detect/1(out_1) -> Latch1/1(in_1)
  loop breaker3/1 -> SampHold?2/2(S/H?)
  loop breaker2/1 -> loop breaker3/1
  Latch1/1(out_1) -> loop breaker2/1
  value(in)/1 -> leading edge detect/1(in_1), trailing edge detect/1(in_1), SampHold?2/1(Input)
  trailing edge detect/1(out_1) -> Variable Transport Delay/1
  SampHold?2/1(output) -> value(out)/1
  stretch/1 -> Product/1
  Product/1 -> Variable Transport Delay/2
  " x/1000"/1 -> Product/2

== system fixlib/Fixation7/Boolify2 ==
  In1 : Inport  Port=1  LatchInput=off
  Abs2 : Abs  SaturateOnIntegerOverflow=on
  direction1 : Subsystem
      mask Type: Sign
      mask Description: y = sign(x)
      mask Help: Sign Function:\n\t\t\ty = 1 if x > 0\n\t\t\ty = 0 if x = 0\n\t\t\ty = -1 if x < 0
      mask Display: plot(-50,-50,50,50,[-50,50],[0,0],[0,0],[-50,50],[-40,0],[-30,-30],[0,40],[30,30])
  Out1 : Outport  InitialOutput=0
  wires:
  direction1/1(out_1) -> Out1/1
  In1/1 -> Abs2/1
  Abs2/1 -> direction1/1(in_1)

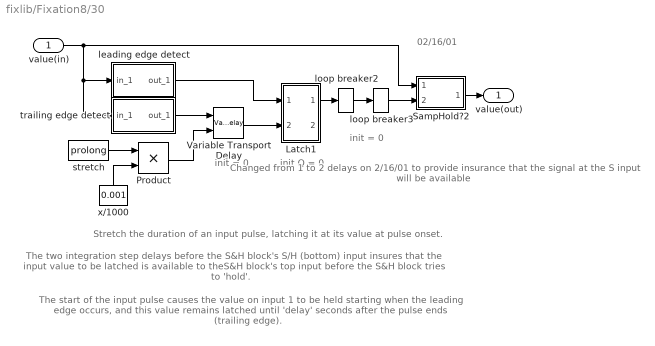
== system fixlib/Fixation8/30  ==
  note: init = 0
  note: init = 0
  note: 02/16/01
  note: The start of the input pulse causes the value on input 1 to be held starting when the leading
      | edge occurs, and this value remains latched until 'delay' seconds after the pulse ends (trailing edge).
  note: The two integration step delays before the S&H block's S/H (bottom) input insures
      | that the input value to be latched is available to theS&H block's top input
      | before the S&H block tries to 'hold'.
  note: Stretch the duration of an input pulse, latching it at its value at pulse onset.
  note: init Q = 0
  note: Changed from 1 to 2 delays
      | on 2/16/01 to provide insurance that
      | the signal at the S input will be available
  value(in) : Inport  Port=1  LatchInput=off
  " x/1000" : Constant  Orientation=up  Value=0.001
  Latch1 : Subsystem  mask(Latch){@1=0}
      mask prompts: @1 "Initial State for Output "Q":"
      mask help: Latch
      mask init:
      | ini=(@1~=0);
      mask Help: Latches the S input.  When S (set) is one, the Q output  becomes one.  The output remains one until the R (reset) input becomes one, forcing the output to zero.  If both R and S are one, the latch will be in an undefined state.
      mask Display: disp('S   Q\n\nR  !Q')
  Product : Product  SaturateOnIntegerOverflow=on  RndMeth=Zero  InputSameDT=on
  SampHold?2 : Subsystem
      mask Display: disp('S=L\nH=H')
  Variable Transport Delay : VariableTransportDelay  MaximumDelay=10
  leading edge detect : Subsystem
      mask Display: disp('Leading\nEdge Det')
  loop breaker2 : Memory
  loop breaker3 : Memory
  stretch : Constant  Value=prolong
  trailing edge detect : Subsystem
      mask Display: disp('Trailing\nEdge Det')
  value(out) : Outport  InitialOutput=0
  wires:
  " x/1000"/1 -> Product/2
  Product/1 -> Variable Transport Delay/2
  stretch/1 -> Product/1
  SampHold?2/1(output) -> value(out)/1
  trailing edge detect/1(out_1) -> Variable Transport Delay/1
  value(in)/1 -> SampHold?2/1(Input), trailing edge detect/1(in_1), leading edge detect/1(in_1)
  Latch1/1(out_1) -> loop breaker2/1
  loop breaker2/1 -> loop breaker3/1
  loop breaker3/1 -> SampHold?2/2(S/H?)
  leading edge detect/1(out_1) -> Latch1/1(in_1)
  Variable Transport Delay/1 -> Latch1/2(in_2)

== system fixlib/Fixation8/Boolify2 ==
  In1 : Inport  Port=1  LatchInput=off
  Abs2 : Abs  SaturateOnIntegerOverflow=on
  direction1 : Subsystem
      mask Type: Sign
      mask Description: y = sign(x)
      mask Help: Sign Function:\n\t\t\ty = 1 if x > 0\n\t\t\ty = 0 if x = 0\n\t\t\ty = -1 if x < 0
      mask Display: plot(-50,-50,50,50,[-50,50],[0,0],[0,0],[-50,50],[-40,0],[-30,-30],[0,40],[30,30])
  Out1 : Outport  InitialOutput=0
  wires:
  Abs2/1 -> direction1/1(in_1)
  In1/1 -> Abs2/1
  direction1/1(out_1) -> Out1/1

== system fixlib/Fixation7/30 /Latch1 ==
  in_1 : Inport  Port=1  LatchInput=off
  in_2 : Inport  Port=2  LatchInput=off
  Demux : Demux  Outputs=2
  Logic : CombinatorialLogic  TruthTable=[0 1;0 1;1 0;0 1;1 0;0 1;1 0;1 0]
  Memory : Memory  Orientation=left  X0=ini
  Mux : Mux  Inputs=3
  out_1 : Outport  InitialOutput=0
  out_2 : Outport  Port=2  InitialOutput=0
  wires:
  Demux/2 -> out_2/1
  Logic/1 -> Demux/1
  Mux/1 -> Logic/1
  Demux/1 -> out_1/1, Memory/1
  Memory/1 -> Mux/1
  in_1/1 -> Mux/2
  in_2/1 -> Mux/3

== system fixlib/Fixation7/30 /SampHold?2 ==
  note: When "S/H?" is LOW, then "Input" is switched directly to the
      | output ("sample").  When "S/H?" is HIGH, the current output is
      | maintained ("hold").
  Input : Inport  Port=1  LatchInput=off
  S/H? : Inport  Port=2  LatchInput=off
  Memory : Memory  Orientation=left
  Sign : Subsystem
      mask Type: Sign
      mask Description: y = sign(x)
      mask Help: Sign Function:\n\t\t\ty = 1 if x > 0\n\t\t\ty = 0 if x = 0\n\t\t\ty = -1 if x < 0
      mask Display: plot(-50,-50,50,50,[-50,50],[0,0],[0,0],[-50,50],[-40,0],[-30,-30],[0,40],[30,30])
  Switch2 : Switch  Threshold=0.5  SaturateOnIntegerOverflow=on  InputSameDT=on
  output : Outport  InitialOutput=0
  wires:
  Memory/1 -> Switch2/1
  Switch2/1 -> output/1, Memory/1
  Input/1 -> Switch2/3
  Sign/1(out_1) -> Switch2/2
  S/H?/1 -> Sign/1(in_1)

== system fixlib/Fixation7/30 /leading edge detect ==
  note: leading edge detection
  in_1 : Inport  Port=1  LatchInput=off
  Abs : Abs  SaturateOnIntegerOverflow=on
  Derivative : Derivative
  Relational Operator : RelationalOperator  Operator===  InputSameDT=on
  Sign : Subsystem
      mask Type: Sign
      mask Description: y = sign(x)
      mask Help: Sign Function:\n\t\t\ty = 1 if x > 0\n\t\t\ty = 0 if x = 0\n\t\t\ty = -1 if x < 0
      mask Display: plot(-50,-50,50,50,[-50,50],[0,0],[0,0],[-50,50],[-40,0],[-30,-30],[0,40],[30,30])
  Threshold 1 : Constant
  out_1 : Outport  InitialOutput=0
  wires:
  Abs/1 -> Derivative/1
  Derivative/1 -> Sign/1(in_1)
  Sign/1(out_1) -> Relational Operator/1
  Threshold 1/1 -> Relational Operator/2
  Relational Operator/1 -> out_1/1
  in_1/1 -> Abs/1

== system fixlib/Fixation7/30 /trailing edge detect ==
  note: trailing edge detection
  note: It is also possible to remove the SIGNUM function
      | and the '==', and replace them with a simple
      | switch with a threshold of (say) 150 or so.
  in_1 : Inport  Port=1  LatchInput=off
  Abs : Abs  SaturateOnIntegerOverflow=on
  Derivative : Derivative
  Relational Operator : RelationalOperator  Operator===  InputSameDT=on
  Sign : Subsystem
      mask Type: Sign
      mask Description: y = sign(x)
      mask Help: Sign Function:\n\t\t\ty = 1 if x > 0\n\t\t\ty = 0 if x = 0\n\t\t\ty = -1 if x < 0
      mask Display: plot(-50,-50,50,50,[-50,50],[0,0],[0,0],[-50,50],[-40,0],[-30,-30],[0,40],[30,30])
  Threshold 1 : Constant  Value=-1
  out_1 : Outport  InitialOutput=0
  wires:
  in_1/1 -> Abs/1
  Relational Operator/1 -> out_1/1
  Threshold 1/1 -> Relational Operator/2
  Sign/1(out_1) -> Relational Operator/1
  Derivative/1 -> Sign/1(in_1)
  Abs/1 -> Derivative/1

== system fixlib/Fixation7/Boolify2/direction1 ==
  in_1 : Inport  Port=1  LatchInput=off
  Constant : Constant  Value=0
  Relational Operator : RelationalOperator  Operator=>  InputSameDT=on
  Relational Operator1 : RelationalOperator  Operator=<  InputSameDT=on
  Sum : Sum  Inputs=+-  SaturateOnIntegerOverflow=on  InputSameDT=on
  out_1 : Outport  InitialOutput=0
  wires:
  Sum/1 -> out_1/1
  Relational Operator/1 -> Sum/1
  Relational Operator1/1 -> Sum/2
  Constant/1 -> Relational Operator/2, Relational Operator1/2
  in_1/1 -> Relational Operator1/1, Relational Operator/1

== system fixlib/Fixation8/30 /Latch1 ==
  in_1 : Inport  Port=1  LatchInput=off
  in_2 : Inport  Port=2  LatchInput=off
  Demux : Demux  Outputs=2
  Logic : CombinatorialLogic  TruthTable=[0 1;0 1;1 0;0 1;1 0;0 1;1 0;1 0]
  Memory : Memory  Orientation=left  X0=ini
  Mux : Mux  Inputs=3
  out_1 : Outport  InitialOutput=0
  out_2 : Outport  Port=2  InitialOutput=0
  wires:
  in_2/1 -> Mux/3
  in_1/1 -> Mux/2
  Memory/1 -> Mux/1
  Demux/1 -> Memory/1, out_1/1
  Mux/1 -> Logic/1
  Logic/1 -> Demux/1
  Demux/2 -> out_2/1

== system fixlib/Fixation8/30 /SampHold?2 ==
  note: When "S/H?" is LOW, then "Input" is switched directly to the
      | output ("sample").  When "S/H?" is HIGH, the current output is
      | maintained ("hold").
  Input : Inport  Port=1  LatchInput=off
  S/H? : Inport  Port=2  LatchInput=off
  Memory : Memory  Orientation=left
  Sign : Subsystem
      mask Type: Sign
      mask Description: y = sign(x)
      mask Help: Sign Function:\n\t\t\ty = 1 if x > 0\n\t\t\ty = 0 if x = 0\n\t\t\ty = -1 if x < 0
      mask Display: plot(-50,-50,50,50,[-50,50],[0,0],[0,0],[-50,50],[-40,0],[-30,-30],[0,40],[30,30])
  Switch2 : Switch  Threshold=0.5  SaturateOnIntegerOverflow=on  InputSameDT=on
  output : Outport  InitialOutput=0
  wires:
  S/H?/1 -> Sign/1(in_1)
  Sign/1(out_1) -> Switch2/2
  Input/1 -> Switch2/3
  Switch2/1 -> Memory/1, output/1
  Memory/1 -> Switch2/1

== system fixlib/Fixation8/30 /leading edge detect ==
  note: leading edge detection
  in_1 : Inport  Port=1  LatchInput=off
  Abs : Abs  SaturateOnIntegerOverflow=on
  Derivative : Derivative
  Relational Operator : RelationalOperator  Operator===  InputSameDT=on
  Sign : Subsystem
      mask Type: Sign
      mask Description: y = sign(x)
      mask Help: Sign Function:\n\t\t\ty = 1 if x > 0\n\t\t\ty = 0 if x = 0\n\t\t\ty = -1 if x < 0
      mask Display: plot(-50,-50,50,50,[-50,50],[0,0],[0,0],[-50,50],[-40,0],[-30,-30],[0,40],[30,30])
  Threshold 1 : Constant
  out_1 : Outport  InitialOutput=0
  wires:
  in_1/1 -> Abs/1
  Relational Operator/1 -> out_1/1
  Threshold 1/1 -> Relational Operator/2
  Sign/1(out_1) -> Relational Operator/1
  Derivative/1 -> Sign/1(in_1)
  Abs/1 -> Derivative/1

== system fixlib/Fixation8/30 /trailing edge detect ==
  note: It is also possible to remove the SIGNUM function
      | and the '==', and replace them with a simple
      | switch with a threshold of (say) 150 or so.
  note: trailing edge detection
  in_1 : Inport  Port=1  LatchInput=off
  Abs : Abs  SaturateOnIntegerOverflow=on
  Derivative : Derivative
  Relational Operator : RelationalOperator  Operator===  InputSameDT=on
  Sign : Subsystem
      mask Type: Sign
      mask Description: y = sign(x)
      mask Help: Sign Function:\n\t\t\ty = 1 if x > 0\n\t\t\ty = 0 if x = 0\n\t\t\ty = -1 if x < 0
      mask Display: plot(-50,-50,50,50,[-50,50],[0,0],[0,0],[-50,50],[-40,0],[-30,-30],[0,40],[30,30])
  Threshold 1 : Constant  Value=-1
  out_1 : Outport  InitialOutput=0
  wires:
  Abs/1 -> Derivative/1
  Derivative/1 -> Sign/1(in_1)
  Sign/1(out_1) -> Relational Operator/1
  Threshold 1/1 -> Relational Operator/2
  Relational Operator/1 -> out_1/1
  in_1/1 -> Abs/1

== system fixlib/Fixation8/Boolify2/direction1 ==
  in_1 : Inport  Port=1  LatchInput=off
  Constant : Constant  Value=0
  Relational Operator : RelationalOperator  Operator=>  InputSameDT=on
  Relational Operator1 : RelationalOperator  Operator=<  InputSameDT=on
  Sum : Sum  Inputs=+-  SaturateOnIntegerOverflow=on  InputSameDT=on
  out_1 : Outport  InitialOutput=0
  wires:
  in_1/1 -> Relational Operator/1, Relational Operator1/1
  Constant/1 -> Relational Operator1/2, Relational Operator/2
  Relational Operator1/1 -> Sum/2
  Relational Operator/1 -> Sum/1
  Sum/1 -> out_1/1

== system fixlib/Fixation7/30 /SampHold?2/Sign ==
  in_1 : Inport  Port=1  LatchInput=off
  Constant : Constant  Value=0
  Relational Operator : RelationalOperator  Operator=>  InputSameDT=on
  Relational Operator1 : RelationalOperator  Operator=<  InputSameDT=on
  Sum : Sum  Inputs=+-  SaturateOnIntegerOverflow=on  InputSameDT=on
  out_1 : Outport  InitialOutput=0
  wires:
  Sum/1 -> out_1/1
  Relational Operator/1 -> Sum/1
  Relational Operator1/1 -> Sum/2
  Constant/1 -> Relational Operator/2, Relational Operator1/2
  in_1/1 -> Relational Operator1/1, Relational Operator/1

== system fixlib/Fixation7/30 /leading edge detect/Sign ==
  in_1 : Inport  Port=1  LatchInput=off
  Constant : Constant  Value=0
  Relational Operator : RelationalOperator  Operator=>  InputSameDT=on
  Relational Operator1 : RelationalOperator  Operator=<  InputSameDT=on
  Sum : Sum  Inputs=+-  SaturateOnIntegerOverflow=on  InputSameDT=on
  out_1 : Outport  InitialOutput=0
  wires:
  in_1/1 -> Relational Operator/1, Relational Operator1/1
  Constant/1 -> Relational Operator1/2, Relational Operator/2
  Relational Operator1/1 -> Sum/2
  Relational Operator/1 -> Sum/1
  Sum/1 -> out_1/1

== system fixlib/Fixation7/30 /trailing edge detect/Sign ==
  in_1 : Inport  Port=1  LatchInput=off
  Constant : Constant  Value=0
  Relational Operator : RelationalOperator  Operator=>  InputSameDT=on
  Relational Operator1 : RelationalOperator  Operator=<  InputSameDT=on
  Sum : Sum  Inputs=+-  SaturateOnIntegerOverflow=on  InputSameDT=on
  out_1 : Outport  InitialOutput=0
  wires:
  Sum/1 -> out_1/1
  Relational Operator/1 -> Sum/1
  Relational Operator1/1 -> Sum/2
  Constant/1 -> Relational Operator/2, Relational Operator1/2
  in_1/1 -> Relational Operator1/1, Relational Operator/1

== system fixlib/Fixation8/30 /SampHold?2/Sign ==
  in_1 : Inport  Port=1  LatchInput=off
  Constant : Constant  Value=0
  Relational Operator : RelationalOperator  Operator=>  InputSameDT=on
  Relational Operator1 : RelationalOperator  Operator=<  InputSameDT=on
  Sum : Sum  Inputs=+-  SaturateOnIntegerOverflow=on  InputSameDT=on
  out_1 : Outport  InitialOutput=0
  wires:
  in_1/1 -> Relational Operator/1, Relational Operator1/1
  Constant/1 -> Relational Operator1/2, Relational Operator/2
  Relational Operator1/1 -> Sum/2
  Relational Operator/1 -> Sum/1
  Sum/1 -> out_1/1

== system fixlib/Fixation8/30 /leading edge detect/Sign ==
  in_1 : Inport  Port=1  LatchInput=off
  Constant : Constant  Value=0
  Relational Operator : RelationalOperator  Operator=>  InputSameDT=on
  Relational Operator1 : RelationalOperator  Operator=<  InputSameDT=on
  Sum : Sum  Inputs=+-  SaturateOnIntegerOverflow=on  InputSameDT=on
  out_1 : Outport  InitialOutput=0
  wires:
  Sum/1 -> out_1/1
  Relational Operator/1 -> Sum/1
  Relational Operator1/1 -> Sum/2
  Constant/1 -> Relational Operator/2, Relational Operator1/2
  in_1/1 -> Relational Operator1/1, Relational Operator/1

== system fixlib/Fixation8/30 /trailing edge detect/Sign ==
  in_1 : Inport  Port=1  LatchInput=off
  Constant : Constant  Value=0
  Relational Operator : RelationalOperator  Operator=>  InputSameDT=on
  Relational Operator1 : RelationalOperator  Operator=<  InputSameDT=on
  Sum : Sum  Inputs=+-  SaturateOnIntegerOverflow=on  InputSameDT=on
  out_1 : Outport  InitialOutput=0
  wires:
  in_1/1 -> Relational Operator/1, Relational Operator1/1
  Constant/1 -> Relational Operator1/2, Relational Operator/2
  Relational Operator1/1 -> Sum/2
  Relational Operator/1 -> Sum/1
  Sum/1 -> out_1/1
